simulink model "DSMLibEasyTest"  (R2016b)
settings: Solver=ode3  StartTime=0.0  StopTime=10  FixedStep=10e-3  RelTol=1e-3
undefined symbols (not defined in the file or in its folder): DFC, FID, sigbuilder_block
libraries: simulink x6, DSMLib x6
settings Model: Creator=Administrator  LastModifiedBy=Administrator
settings OptimizationCC: DefaultParameterBehavior=Inlined
settings DebuggingCC: ParameterTunabilityLossMsg=error
settings RTWCC: SystemTargetFile=ert.tlc  TemplateMakefile=ert_default_tmf  Description=Embedded Coder  GenerateReport=on  IncludeHyperlinkInReport=on  LaunchReport=on  GenerateTraceInfo=on  GenerateTraceReport=on  GenerateTraceReportSl=on  GenerateTraceReportSf=on  GenerateTraceReportEml=on
settings RTWCC: CustomInclude=|
  | C:\MatlabWS\motorcontrol\sfun
  | C:\MatlabWS\motorcontrol\sfun\DSM
settings RTWCC: CustomSource=|
  | C:/MatlabWS/motorcontrol/sfun/DSM/core_env.h
  | C:/MatlabWS/motorcontrol/sfun/DSM/DCC_Diag_conf.XML
  | C:/MatlabWS/motorcontrol/sfun/DSM/ddrc_conf.c
  | C:/MatlabWS/motorcontrol/sfun/DSM/ddrc_dat.h
  | C:/MatlabWS/motorcontrol/sfun/DSM/ddrc_get_status.c
  | C:/MatlabWS/motorcontrol/sfun/DSM/ddrc_init.c
  | C:/MatlabWS/motorcontrol/sfun/DSM/ddrc_no_deb.c
  | C:/MatlabWS/motorcontrol/sfun/DSM/ddrc_pub.h
  | C:/MatlabWS/motorcontrol/sfun/DSM/ddrc_reset.c
  | C:/MatlabWS/motorcontrol/sfun/DSM/ddrc_ti_row_sm.c
  | C:/MatlabWS/motorcontrol/sfun/DSM/dfc_auto_conf.c
  | C:/MatlabWS/motorcontrol/sfun/DSM/dfc_auto_conf.h
  | C:/MatlabWS/motorcontrol/sfun/DSM/dfc_conf.c
  | C:/MatlabWS/motorcontrol/sfun/DSM/dfc_dat.h
  | C:/MatlabWS/motorcontrol/sfun/DSM/dfc_init.c
  | C:/MatlabWS/motorcontrol/sfun/DSM/dfc_pub.h
  | C:/MatlabWS/motorcontrol/sfun/DSM/dfc_report.c
  | C:/MatlabWS/motorcontrol/sfun/DSM/dfes_check_state.c
  | C:/MatlabWS/motorcontrol/sfun/DSM/dfes_conf.c
  | C:/MatlabWS/motorcontrol/sfun/DSM/dfes_create_entry.c
  | C:/MatlabWS/motorcontrol/sfun/DSM/dfes_dat.h
  | C:/MatlabWS/motorcontrol/sfun/DSM/dfes_entry_prio.c
  | C:/MatlabWS/motorcontrol/sfun/DSM/dfes_hash.c
  | C:/MatlabWS/motorcontrol/sfun/DSM/dfes_init.c
  | C:/MatlabWS/motorcontrol/sfun/DSM/Dfes_pub.h
  | C:/MatlabWS/motorcontrol/sfun/DSM/dfes_report.c
  | C:/MatlabWS/motorcontrol/sfun/DSM/dfes_scan_order.c
  | C:/MatlabWS/motorcontrol/sfun/DSM/dinh_auto_conf.c
  | C:/MatlabWS/motorcontrol/sfun/DSM/dinh_auto_conf.h
  | C:/MatlabWS/motorcontrol/sfun/DSM/dinh_conf.c
  | C:/MatlabWS/motorcontrol/sfun/DSM/dinh_dat.h
  | C:/MatlabWS/motorcontrol/sfun/DSM/dinh_getpermission.c
  | C:/MatlabWS/motorcontrol/sfun/DSM/dinh_init.c
  | C:/MatlabWS/motorcontrol/sfun/DSM/dinh_pub.h
  | C:/MatlabWS/motorcontrol/sfun/DSM/dinh_upt_dfc.c
  | C:/MatlabWS/motorcontrol/sfun/DSM/DSM.bat
  | C:/MatlabWS/motorcontrol/sfun/DSM/dsm.h
  | C:/MatlabWS/motorcontrol/sfun/DSM/dsm_dat.c
  | C:/MatlabWS/motorcontrol/sfun/DSM/dsm_debCheck.c
  | C:/MatlabWS/motorcontrol/sfun/DSM/dsm_process.pl
  | C:/MatlabWS/motorcontrol/sfun/DSM/dsmaux_prot.h
  | C:/MatlabWS/motorcontrol/sfun/DSM/Dsmaux_syc_reinit.c
  | C:/MatlabWS/motorcontrol/sfun/DSM/ppctypes.h
  | C:/MatlabWS/motorcontrol/sfun/DSM/Srvb_adapter.h
  | C:/MatlabWS/motorcontrol/sfun/C2SfunShell_DSM.c
settings CodeAppCC: ForceParamTrailComments=on  IgnoreCustomStorageClasses=off  OperatorAnnotations=on  SimulinkDataObjDesc=on  SFDataObjDesc=on  MATLABFcnDesc=on  InsertBlockDesc=on  MATLABSourceComments=on
settings ERTTargetCC: TargetLangStandard=C99 (ISO)  GenerateSampleERTMain=on  InlinedParameterPlacement=NonHierarchical  ERTCustomFileTemplate=example_file_process.tlc

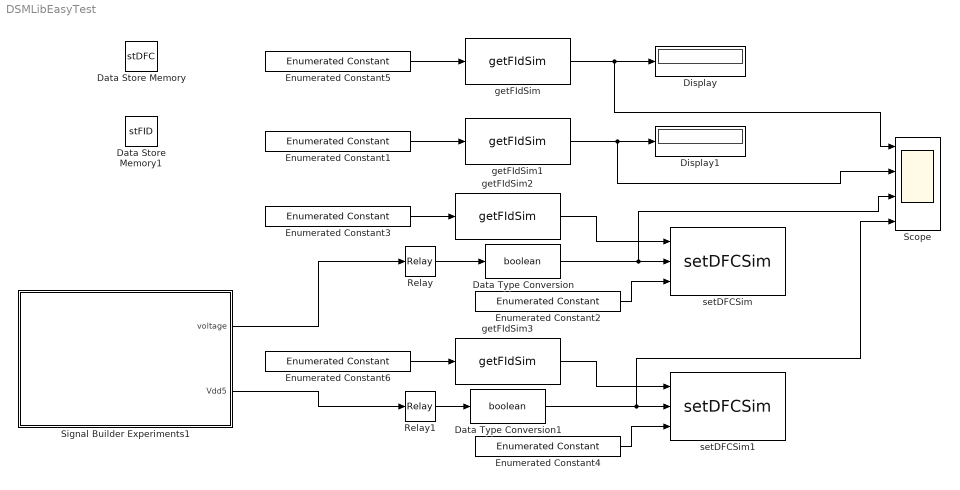
== system DSMLibEasyTest ==
  Data Store Memory : DataStoreMemory  DataStoreName=stDFC  ReadBeforeWriteMsg=warning  WriteAfterWriteMsg=warning  WriteAfterReadMsg=warning  InitialValue=zeros(1,512)  ShowAdditionalParam=off  OutDataTypeStr=boolean
  Data Store Memory1 : DataStoreMemory  DataStoreName=stFID  ReadBeforeWriteMsg=warning  WriteAfterWriteMsg=warning  WriteAfterReadMsg=warning  InitialValue=ones(1,512)  ShowAdditionalParam=off  OutDataTypeStr=boolean
  Data Type Conversion : DataTypeConversion  OutDataTypeStr=boolean
  Data Type Conversion1 : DataTypeConversion  OutDataTypeStr=boolean
  Display : Display
  Display1 : Display
  Enumerated Constant1 : simulink/Sources/Enumerated Constant  OutDataTypeStr=Enum: FID  Value=FID.SnduVdd5g1Under  SampleTime=inf
  Enumerated Constant2 : simulink/Sources/Enumerated Constant  OutDataTypeStr=Enum: DFC  Value=DFC.uDclinkOver  SampleTime=inf
  Enumerated Constant3 : simulink/Sources/Enumerated Constant  OutDataTypeStr=Enum: FID  Value=FID.DiaguDclinkOver  SampleTime=inf
  Enumerated Constant4 : simulink/Sources/Enumerated Constant  OutDataTypeStr=Enum: DFC  Value=DFC.uVdd5g1Under  SampleTime=inf
  Enumerated Constant5 : simulink/Sources/Enumerated Constant  OutDataTypeStr=Enum: FID  Value=FID.SnduDclinkOver  SampleTime=inf
  Enumerated Constant6 : simulink/Sources/Enumerated Constant  OutDataTypeStr=Enum: FID  Value=FID.DiaguVdd5g1Under  SampleTime=inf
  Relay : Relay  OnSwitchValue=410  OffSwitchValue=380
  Relay1 : Relay  OnSwitchValue=4.5  OffSwitchValue=4.2  OnOutputValue=0  OffOutputValue=1
  Scope : Scope  NumInputPorts=4
  Signal Builder Experiments1 : Subsystem  Tag=STV Subsys  LoadFcn=sigbuilder_block('load',[6 61.5 1012.5 405.75 ]);  StartFcn=sigbuilder_block('start');  StopFcn=sigbuilder_block('stop');  ClipboardFcn=sigbuilder_block('clipboard');  mask(Sigbuilder block){tuvar=[0:10]}
      mask help: Sigbuilder GUI
      mask init:
      | if ~strcmp(get_param(bdroot(gcbh),'SimulationStatus'),'stopped') tuvar = sigbuilder_block('maskInit'); end
      settings: CopyFcn=sigbuilder_block('copy');  DeleteFcn=sigbuilder_block('delete');  ModelCloseFcn=sigbuilder_block('modelClose');  PreSaveFcn=sigbuilder_block('preSave');  PauseFcn=sigbuilder_block('pause')  ContinueFcn=sigbuilder_block('continue')  NameChangeFcn=sigbuilder_block('namechange');  OpenFcn=sigbuilder_block('open',[6 61.5 1012.5 405.75 ]);  CloseFcn=sigbuilder_block('close');  MinAlgLoopOccurrences=on
      mask Display: plot(0, 0, 100, 100,[2, 2, 32, 32, 2], [68, 8, 8, 68, 68],[32, 2], [38, 38], [32, 19, 2],[53, 60, 44], [32, 17, 17, 2],[16, 16, 31, 31]);txt = getActiveGroup(gcbh);text(2, 100, txt,'verticalAlignment', 'top');
  getFIdSim{,1..3} (4 alike) : DSMLib/getFIdSim
  setDFCSim : DSMLib/setDFCSim
  setDFCSim1 : DSMLib/setDFCSim
  wires:
  Enumerated Constant5/1 -> getFIdSim/1
  getFIdSim/1 -> Scope/1, Display/1
  Enumerated Constant1/1 -> getFIdSim1/1
  getFIdSim1/1 -> Scope/2, Display1/1
  Enumerated Constant3/1 -> getFIdSim2/1
  Signal Builder Experiments1/1(voltage) -> Relay/1
  Enumerated Constant2/1 -> setDFCSim/3
  Relay/1 -> Data Type Conversion/1
  Enumerated Constant6/1 -> getFIdSim3/1
  Signal Builder Experiments1/2(Vdd5) -> Relay1/1
  Enumerated Constant4/1 -> setDFCSim1/3
  Relay1/1 -> Data Type Conversion1/1
  getFIdSim2/1 -> setDFCSim/1
  getFIdSim3/1 -> setDFCSim1/1
  Data Type Conversion/1 -> Scope/3, setDFCSim/2
  Data Type Conversion1/1 -> Scope/4, setDFCSim1/2

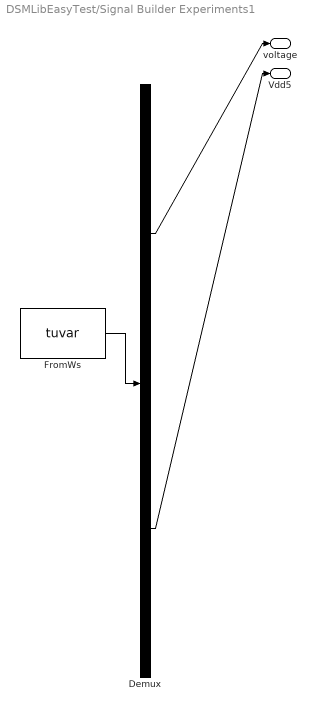
== system DSMLibEasyTest/Signal Builder Experiments1 ==
  Demux : Demux  Tag=STV Demux  Outputs=2
  FromWs : FromWorkspace  Tag=STV FromWs  VariableName=tuvar  SampleTime=0.01  OutputAfterFinalValue=Holding final value
      SigBuilderData=|
      | common.afterFinalStr = 'Hold final value'
      | common.sampleTime = '0.01'
      | dataSet.timeRange = [0 10]
      | dataSet.name = 'Hi Velocity'
      | sbobj.Groups.Name = 'Hi Velocity'
      | sbobj.Groups.Signals(1).Name = 'voltage'
      | sbobj.Groups.Signals(1).XData = [0 3 8 10]
      | sbobj.Groups.Signals(1).YData = [360 415 600 90]
      | sbobj.Groups.Signals(2).Name = 'Vdd5'
      | sbobj.Groups.Signals(2).XData = [0 5.46 5.46 8 10]
      | sbobj.Groups.Signals(2).YData = [-0.5 -0.5 5 3.85 0]
  voltage : Outport  Tag=STV Outport
  Vdd5 : Outport  Tag=STV Outport  Port=2
  wires:
  FromWs/1 -> Demux/1
  Demux/1 -> voltage/1
  Demux/2 -> Vdd5/1
